simulink model "jointsControl"  (Simulink 9.1)
settings: Solver=FixedStepDiscrete  StartTime=0.0  StopTime=Config.SIMULATION_TIME  FixedStep=Config.tStep  RelTol=1e-3  EnableMultiTasking=on
PostLoadFcn:
  | %% Try to open the static GUI
  | try
  | 
  |     staticGUI = simulinkStaticGUI;
  | 
  | end
InitFcn:
  | %% initialize the simulation
  | cd(fileparts(which(bdroot)));
  | initJointsControl;
  | 
  | %% Try to edit the GUI (the user may have already closed it)
  | try
  | 
  |     %% Update Start Button
  |     set(sl_synch_handles.startButton,'Backgroundcolor',[0.0,1.0,0.0]);
  |     set(sl_synch_handles.startButton,'Enable','on');
  | 
  | end
StartFcn:
  | %% Try to edit the GUI (the user may have already closed it)
  | try
  | 
  |     %% Update Start Button
  |     set(sl_synch_handles.startButton,'Backgroundcolor',[0.8,0.8,0.8]);
  |     set(sl_synch_handles.startButton,'Enable','off');
  | 
  |     %% Update Compile Button
  |     set(sl_synch_handles.compileButton,'Backgroundcolor',[0.8,0.8,0.8]);
  |     set(sl_synch_handles.compileButton,'Enable','off');
  | 
  |     %% Update Exit Button
  |     set(sl_synch_handles.exitButton,'Backgroundcolor',[0.8,0.8,0.8]);
  |     set(sl_synch_handles.exitButton,'Enable','off');
  | 
  | end
StopFcn:
  | %% stop the simulation
  | cd(fileparts(which(bdroot)));
  | stopJointsControl;
  | 
  | %% Try to edit the GUI (the user may have already closed it)
  | try
  | 
  |     %% Update Compile Button
  |     set(sl_synch_handles.compileButton,'Backgroundcolor',[1.0,0.6,0.0]);
  |     set(sl_synch_handles.compileButton,'Enable','on');
  | 
  |     %% Update Exit Button
  |     set(sl_synch_handles.exitButton,'Backgroundcolor',[0.0,1.0,1.0]);
  |     set(sl_synch_handles.exitButton,'Enable','on');
  | 
  | end
undefined symbols (not defined in the file): Config, KD, KP, Ref, ROBOT_DOF, Sat
libraries: WBToolboxLibrary x12
CloseFcn:
  | %% Try to close the GUI (the user might have already closed it)
  | try
  | 
  |     close(simulinkStaticGUI)
  | 
  | end
settings Model: SuppressorTable=22 serialization::archive 11 0 6 0 0 0 1 0  Creator=daniele  LastModifiedBy=icub
settings DataIOCC: LimitDataPoints=on  SignalLoggingSaveFormat=ModelDataLogs
settings DebuggingCC: UnderspecifiedInitializationDetection=Simplified  MergeDetectMultiDrivingBlocksExec=error  SolverPrmCheckMsg=warning  MultiTaskDSMMsg=warning  MultiTaskCondExecSysMsg=none  AllowSymbolicDim=off  StrictBusMsg=ErrorOnBusTreatedAsVector
settings GRTTargetCC: GeneratePreprocessorConditionals=Disable all  CombineOutputUpdateFcns=on  GRTInterface=off

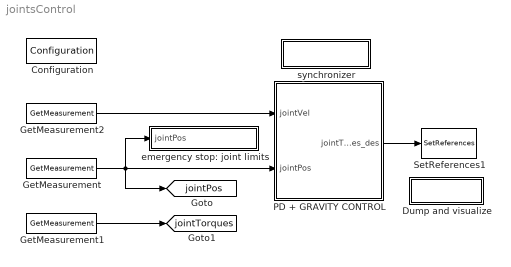
== system jointsControl ==
  Configuration : WBToolboxLibrary/Utilities/Configuration  ConfigSource=Workspace  ConfigObject='WBTConfigRobot'
      settings: SourceProductName=WholeBodyToolbox
  Dump and visualize : Subsystem
      mask Display: disp('VISUALIZER')
  GetMeasurement : WBToolboxLibrary/States/GetMeasurement  measuredType=Joints Position
      settings: SourceProductName=WholeBodyToolbox
  GetMeasurement1 : WBToolboxLibrary/States/GetMeasurement  measuredType=Joints Torque
      settings: SourceProductName=WholeBodyToolbox
  GetMeasurement2 : WBToolboxLibrary/States/GetMeasurement  measuredType=Joints Velocity
      settings: SourceProductName=WholeBodyToolbox
  PD + GRAVITY CONTROL : Subsystem
  SetReferences1 : WBToolboxLibrary/Actuators/SetReferences  controlType=Torque  refSpeed=50  refAcceleration=1000000*(pi/180)
      settings: SourceProductName=WholeBodyToolbox
  emergency stop: joint limits : Subsystem
      mask Display: disp('EMERGENCY STOP')
  synchronizer : Subsystem
      mask Display: disp('SYNCHRONIZER')
  tag scope: jointPos=global, jointTorques=global
  wires:
  GetMeasurement/1 -> [jointPos], emergency stop: joint limits/1(jointPos), PD + GRAVITY CONTROL/2(jointPos)
  PD + GRAVITY CONTROL/1(jointTorques_des) -> SetReferences1/1
  GetMeasurement2/1 -> PD + GRAVITY CONTROL/1(jointVel)
  GetMeasurement1/1 -> [jointTorques]

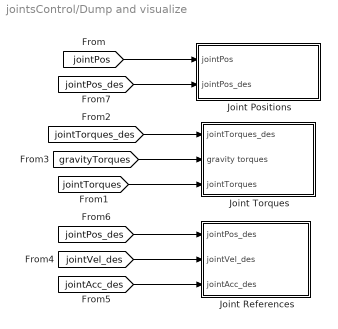
== system jointsControl/Dump and visualize ==
  Joint Positions : Subsystem
  Joint References : Subsystem
  Joint Torques : Subsystem
  wires:
  [jointTorques] -> Joint Torques/3(jointTorques)
  [gravityTorques] -> Joint Torques/2(gravity torques)
  [jointTorques_des] -> Joint Torques/1(jointTorques_des)
  [jointPos] -> Joint Positions/1(jointPos)
  [jointPos_des] -> Joint References/1(jointPos_des)
  [jointVel_des] -> Joint References/2(jointVel_des)
  [jointAcc_des] -> Joint References/3(jointAcc_des)
  [jointPos_des] -> Joint Positions/2(jointPos_des)

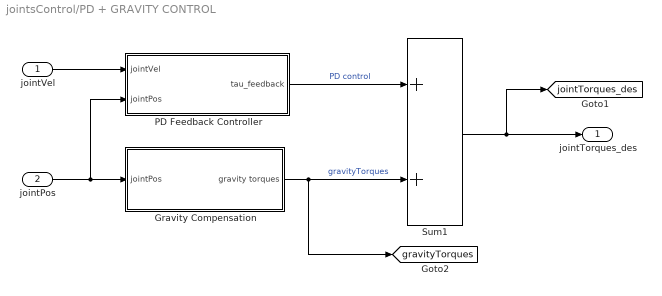
== system jointsControl/PD + GRAVITY CONTROL ==
  jointVel : Inport
  jointPos : Inport  Port=2
  Gravity Compensation : Subsystem
  PD Feedback Controller : Subsystem
  Sum1 : Sum
  jointTorques_des : Outport
  tag scope: gravityTorques=global, jointTorques_des=global
  wires:
  jointPos/1 -> PD Feedback Controller/2(jointPos), Gravity Compensation/1(jointPos)
  jointVel/1 -> PD Feedback Controller/1(jointVel)
  Sum1/1 -> [jointTorques_des], jointTorques_des/1
  Gravity Compensation/1(gravity torques) -> [gravityTorques], Sum1/2  "gravityTorques"
  PD Feedback Controller/1(tau_feedback) -> Sum1/1  "PD control"

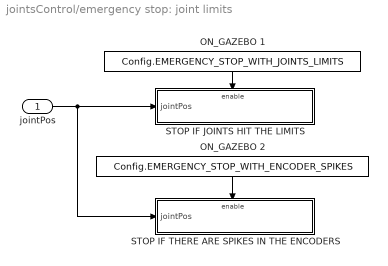
== system jointsControl/emergency stop: joint limits ==
  jointPos : Inport
  ON_GAZEBO 1 : Constant  Value=Config.EMERGENCY_STOP_WITH_JOINTS_LIMITS
  ON_GAZEBO 2 : Constant  Value=Config.EMERGENCY_STOP_WITH_ENCODER_SPIKES
  STOP IF JOINTS HIT THE LIMITS : Subsystem
  STOP IF THERE ARE SPIKES IN THE ENCODERS : Subsystem
  wires:
  ON_GAZEBO 1/1 -> STOP IF JOINTS HIT THE LIMITS/Enable
  jointPos/1 -> STOP IF THERE ARE SPIKES IN THE ENCODERS/1(jointPos), STOP IF JOINTS HIT THE LIMITS/1(jointPos)
  ON_GAZEBO 2/1 -> STOP IF THERE ARE SPIKES IN THE ENCODERS/Enable

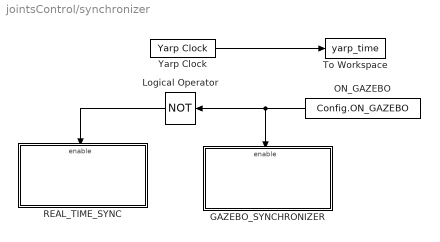
== system jointsControl/synchronizer ==
  GAZEBO_SYNCHRONIZER : Subsystem
  Logical Operator : Logic  Operator=NOT  AllPortsSameDT=off  OutDataTypeStr=boolean
  "ON_GAZEBO " : Constant  Value=Config.ON_GAZEBO
  REAL_TIME_SYNC : Subsystem
  To Workspace : ToWorkspace  VariableName=yarp_time  SaveFormat=Structure With Time  SampleTime=-1
  Yarp Clock : WBToolboxLibrary/Utilities/Yarp Clock
      settings: SourceProductName=WholeBodyToolbox
  wires:
  Logical Operator/1 -> REAL_TIME_SYNC/Enable
  "ON_GAZEBO "/1 -> GAZEBO_SYNCHRONIZER/Enable, Logical Operator/1
  Yarp Clock/1 -> To Workspace/1

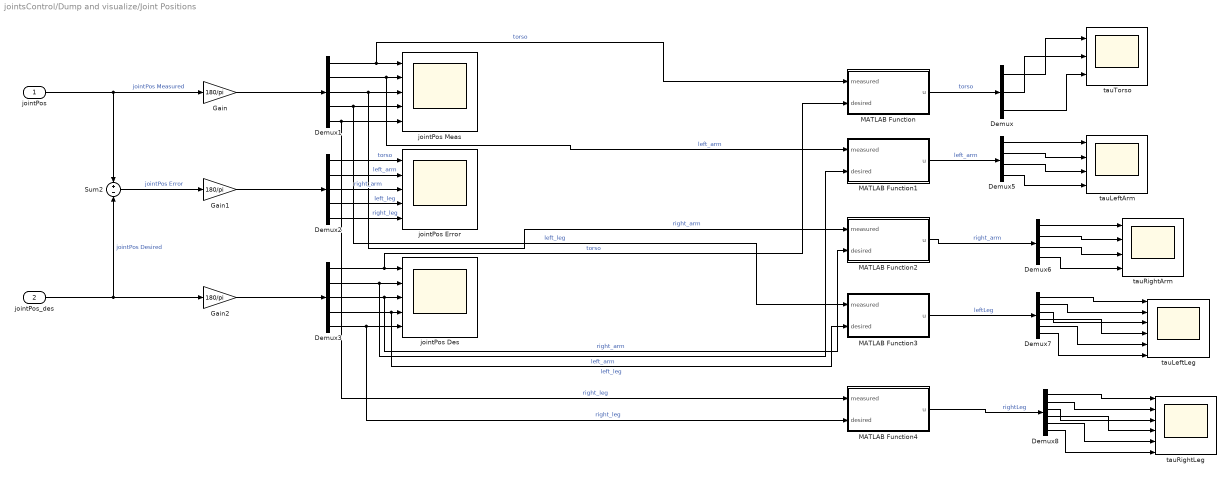
== system jointsControl/Dump and visualize/Joint Positions ==
  jointPos : Inport
  jointPos_des : Inport  Port=2
  Demux : Demux  Outputs=[2 2 2]
  Demux1 : Demux  Outputs=Config.numOfJointsForEachControlboard
  Demux2 : Demux  Outputs=Config.numOfJointsForEachControlboard
  Demux3 : Demux  Outputs=Config.numOfJointsForEachControlboard
  Demux5 : Demux  Outputs=[2 2 2 2]
  Demux6 : Demux  Outputs=[2 2 2 2]
  Demux7 : Demux  Outputs=[2 2 2 2 2 2]
  Demux8 : Demux  Outputs=[2 2 2 2 2 2]
  Gain : Gain  Gain=180/pi
  Gain1 : Gain  Gain=180/pi
  Gain2 : Gain  Gain=180/pi
  MATLAB Function : MATLAB Function  TreatAsAtomicUnit=on
  MATLAB Function1 : MATLAB Function  TreatAsAtomicUnit=on
  MATLAB Function2 : MATLAB Function  TreatAsAtomicUnit=on
  MATLAB Function3 : MATLAB Function  TreatAsAtomicUnit=on
  MATLAB Function4 : MATLAB Function  TreatAsAtomicUnit=on
  Sum2 : Sum  Inputs=+|-
  jointPos Des : Scope  NumInputPorts=5
  jointPos Error : Scope  NumInputPorts=5
  jointPos Meas : Scope  NumInputPorts=5
  tauLeftArm : Scope  NumInputPorts=4
  tauLeftLeg : Scope  NumInputPorts=6
  tauRightArm : Scope  NumInputPorts=4
  tauRightLeg : Scope  NumInputPorts=6
  tauTorso : Scope  NumInputPorts=3
  wires:
  jointPos/1 -> Sum2/1, Gain/1  "jointPos Measured"
  Demux1/2 -> MATLAB Function1/1(measured), jointPos Meas/2  "left_arm"
  Demux1/4 -> MATLAB Function3/1(measured), jointPos Meas/4  "left_leg"
  Demux1/3 -> MATLAB Function2/1(measured), jointPos Meas/3  "right_arm"
  Demux1/5 -> MATLAB Function4/1(measured), jointPos Meas/5  "right_leg"
  Demux2/1 -> jointPos Error/1  "torso"
  Demux2/2 -> jointPos Error/2  "left_arm"
  Demux2/4 -> jointPos Error/4  "left_leg"
  Demux2/3 -> jointPos Error/3  "right_arm"
  Demux2/5 -> jointPos Error/5  "right_leg"
  Sum2/1 -> Gain1/1  "jointPos Error"
  Demux3/1 -> MATLAB Function/2(desired), jointPos Des/1  "torso"
  Demux3/2 -> MATLAB Function1/2(desired), jointPos Des/2  "left_arm"
  Demux3/4 -> MATLAB Function3/2(desired), jointPos Des/4  "left_leg"
  Demux3/3 -> MATLAB Function2/2(desired), jointPos Des/3  "right_arm"
  jointPos_des/1 -> Gain2/1, Sum2/2  "jointPos Desired"
  Demux3/5 -> MATLAB Function4/2(desired), jointPos Des/5  "right_leg"
  Gain/1 -> Demux1/1
  Gain1/1 -> Demux2/1
  Gain2/1 -> Demux3/1
  MATLAB Function4/1(u) -> Demux8/1  "rightLeg"
  Demux5/1 -> tauLeftArm/1
  Demux7/3 -> tauLeftLeg/3
  Demux7/4 -> tauLeftLeg/4
  Demux7/5 -> tauLeftLeg/5
  Demux5/2 -> tauLeftArm/2
  Demux7/1 -> tauLeftLeg/1
  MATLAB Function/1(u) -> Demux/1  "torso"
  Demux6/2 -> tauRightArm/2
  Demux8/4 -> tauRightLeg/4
  Demux6/3 -> tauRightArm/3
  Demux5/4 -> tauLeftArm/4
  Demux1/1 -> MATLAB Function/1(measured), jointPos Meas/1  "torso"
  Demux6/1 -> tauRightArm/1
  MATLAB Function2/1(u) -> Demux6/1  "right_arm"
  Demux/1 -> tauTorso/1
  Demux7/6 -> tauLeftLeg/6
  Demux/2 -> tauTorso/2
  Demux8/1 -> tauRightLeg/1
  Demux6/4 -> tauRightArm/4
  Demux5/3 -> tauLeftArm/3
  Demux/3 -> tauTorso/3
  Demux8/6 -> tauRightLeg/6
  Demux8/5 -> tauRightLeg/5
  MATLAB Function3/1(u) -> Demux7/1  "leftLeg"
  Demux7/2 -> tauLeftLeg/2
  Demux8/2 -> tauRightLeg/2
  MATLAB Function1/1(u) -> Demux5/1  "left_arm"
  Demux8/3 -> tauRightLeg/3

== system jointsControl/Dump and visualize/Joint References ==
  jointPos_des : Inport
  jointVel_des : Inport  Port=2
  jointAcc_des : Inport  Port=3
  Visualize References : Scope  NumInputPorts=3
  wires:
  jointAcc_des/1 -> Visualize References/3
  jointVel_des/1 -> Visualize References/2
  jointPos_des/1 -> Visualize References/1

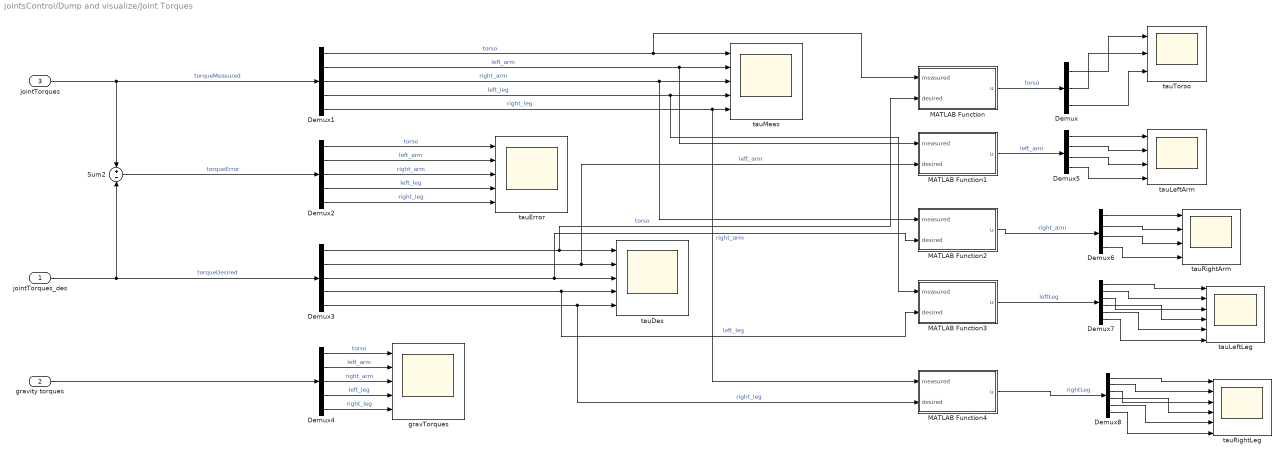
== system jointsControl/Dump and visualize/Joint Torques ==
  jointTorques_des : Inport
  gravity torques : Inport  Port=2
  jointTorques : Inport  Port=3
  Demux : Demux  Outputs=[2 2 2]
  Demux{1..4} (4 alike) : Demux  Outputs=Config.numOfJointsForEachControlboard
  Demux5 : Demux  Outputs=[2 2 2 2]
  Demux6 : Demux  Outputs=[2 2 2 2]
  Demux7 : Demux  Outputs=[2 2 2 2 2 2]
  Demux8 : Demux  Outputs=[2 2 2 2 2 2]
  MATLAB Function : MATLAB Function  TreatAsAtomicUnit=on
  MATLAB Function1 : MATLAB Function  TreatAsAtomicUnit=on
  MATLAB Function2 : MATLAB Function  TreatAsAtomicUnit=on
  MATLAB Function3 : MATLAB Function  TreatAsAtomicUnit=on
  MATLAB Function4 : MATLAB Function  TreatAsAtomicUnit=on
  Sum2 : Sum  Inputs=+|-
  gravTorques : Scope  NumInputPorts=5
  tauDes : Scope  NumInputPorts=5
  tauError : Scope  NumInputPorts=5
  tauLeftArm : Scope  NumInputPorts=4
  tauLeftLeg : Scope  NumInputPorts=6
  tauMeas : Scope  NumInputPorts=5
  tauRightArm : Scope  NumInputPorts=4
  tauRightLeg : Scope  NumInputPorts=6
  tauTorso : Scope  NumInputPorts=3
  wires:
  gravity torques/1 -> Demux4/1
  jointTorques/1 -> Demux1/1, Sum2/1  "torqueMeasured"
  Demux1/1 -> MATLAB Function/1(measured), tauMeas/1  "torso"
  Demux1/2 -> MATLAB Function1/1(measured), tauMeas/2  "left_arm"
  Demux1/4 -> MATLAB Function3/1(measured), tauMeas/4  "left_leg"
  Demux1/3 -> MATLAB Function2/1(measured), tauMeas/3  "right_arm"
  Demux1/5 -> MATLAB Function4/1(measured), tauMeas/5  "right_leg"
  Demux2/1 -> tauError/1  "torso"
  Demux2/2 -> tauError/2  "left_arm"
  Demux2/4 -> tauError/4  "left_leg"
  Demux2/3 -> tauError/3  "right_arm"
  Demux2/5 -> tauError/5  "right_leg"
  Sum2/1 -> Demux2/1  "torqueError"
  Demux3/1 -> MATLAB Function/2(desired), tauDes/1  "torso"
  Demux3/2 -> MATLAB Function1/2(desired), tauDes/2  "left_arm"
  Demux3/4 -> MATLAB Function3/2(desired), tauDes/4  "left_leg"
  Demux3/3 -> MATLAB Function2/2(desired), tauDes/3  "right_arm"
  jointTorques_des/1 -> Demux3/1, Sum2/2  "torqueDesired"
  Demux3/5 -> MATLAB Function4/2(desired), tauDes/5  "right_leg"
  Demux4/1 -> gravTorques/1  "torso"
  Demux4/2 -> gravTorques/2  "left_arm"
  Demux4/4 -> gravTorques/4  "left_leg"
  Demux4/3 -> gravTorques/3  "right_arm"
  Demux4/5 -> gravTorques/5  "right_leg"
  MATLAB Function/1(u) -> Demux/1  "torso"
  Demux/1 -> tauTorso/1
  Demux/2 -> tauTorso/2
  Demux/3 -> tauTorso/3
  MATLAB Function1/1(u) -> Demux5/1  "left_arm"
  Demux5/1 -> tauLeftArm/1
  Demux5/2 -> tauLeftArm/2
  Demux5/3 -> tauLeftArm/3
  Demux5/4 -> tauLeftArm/4
  Demux6/4 -> tauRightArm/4
  Demux6/3 -> tauRightArm/3
  Demux6/2 -> tauRightArm/2
  Demux6/1 -> tauRightArm/1
  MATLAB Function2/1(u) -> Demux6/1  "right_arm"
  MATLAB Function3/1(u) -> Demux7/1  "leftLeg"
  Demux7/1 -> tauLeftLeg/1
  Demux7/2 -> tauLeftLeg/2
  Demux7/3 -> tauLeftLeg/3
  Demux7/4 -> tauLeftLeg/4
  Demux7/5 -> tauLeftLeg/5
  Demux7/6 -> tauLeftLeg/6
  Demux8/6 -> tauRightLeg/6
  Demux8/5 -> tauRightLeg/5
  Demux8/4 -> tauRightLeg/4
  Demux8/3 -> tauRightLeg/3
  Demux8/2 -> tauRightLeg/2
  Demux8/1 -> tauRightLeg/1
  MATLAB Function4/1(u) -> Demux8/1  "rightLeg"

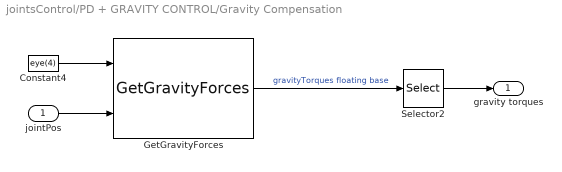
== system jointsControl/PD + GRAVITY CONTROL/Gravity Compensation ==
  jointPos : Inport
  Constant4 : Constant  Value=eye(4)
  GetGravityForces : WBToolboxLibrary/Model/Dynamics/GetGravityForces
      settings: SourceProductName=WholeBodyToolbox
  Selector2 : Selector  InputPortWidth=ROBOT_DOF+6  IndexOptions=Index vector (dialog)  Indices=[7:ROBOT_DOF+6]  OutputSizes=1
  gravity torques : Outport
  wires:
  Selector2/1 -> gravity torques/1
  Constant4/1 -> GetGravityForces/1
  jointPos/1 -> GetGravityForces/2
  GetGravityForces/1 -> Selector2/1  "gravityTorques floating base"

== system jointsControl/PD + GRAVITY CONTROL/PD Feedback Controller ==
  jointVel : Inport
  jointPos : Inport  Port=2
  PD Controller : Subsystem
  Reference Generator : Subsystem
  tau_feedback : Outport
  wires:
  jointVel/1 -> PD Controller/4(jointVel)
  jointPos/1 -> Reference Generator/1(jointPos), PD Controller/5(jointPos)
  PD Controller/1(tau_feedback) -> tau_feedback/1
  Reference Generator/1(Ms*jointAcc_des) -> PD Controller/1(Ms*jointAcc_des)
  Reference Generator/2(jointPos_des) -> PD Controller/2(jointPos_des)
  Reference Generator/3(jointVel_des) -> PD Controller/3(jointVel_des)

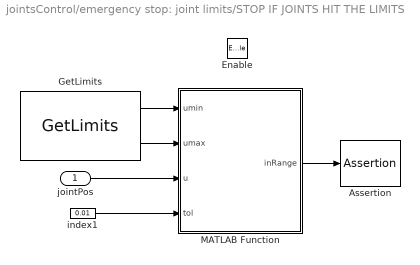
== system jointsControl/emergency stop: joint limits/STOP IF JOINTS HIT THE LIMITS ==
  jointPos : Inport
  Enable : EnablePort
  Assertion : Assertion
  GetLimits : WBToolboxLibrary/States/GetLimits  limitsSource=ControlBoard  limitsType=Position
      settings: SourceProductName=WholeBodyToolbox
  MATLAB Function : MATLAB Function  TreatAsAtomicUnit=on
  index1 : Constant  Value=0.01  VectorParams1D=off
  wires:
  jointPos/1 -> MATLAB Function/3(u)
  MATLAB Function/1(inRange) -> Assertion/1
  GetLimits/1 -> MATLAB Function/1(umin)
  GetLimits/2 -> MATLAB Function/2(umax)
  index1/1 -> MATLAB Function/4(tol)

== system jointsControl/emergency stop: joint limits/STOP IF THERE ARE SPIKES IN THE ENCODERS ==
  jointPos : Inport
  Enable : EnablePort
  Assertion : Assertion
  MATLAB Function : MATLAB Function  TreatAsAtomicUnit=on
  index1 : Constant  Value=Sat.maxJointsPositionDelta  VectorParams1D=off
  wires:
  jointPos/1 -> MATLAB Function/1(u)
  MATLAB Function/1(noSpikes) -> Assertion/1
  index1/1 -> MATLAB Function/2(delta_u_max)

== system jointsControl/synchronizer/GAZEBO_SYNCHRONIZER ==
  Enable : EnablePort
  Simulator Synchronizer : WBToolboxLibrary/Utilities/Simulator Synchronizer  period=Config.tStep  serverPortName='/clock/rpc'  clientPortName='/WBT_synchronizer/rpc:o'
      settings: SourceProductName=WholeBodyToolbox

== system jointsControl/synchronizer/REAL_TIME_SYNC ==
  Enable : EnablePort
  Real Time Synchronizer : WBToolboxLibrary/Utilities/Real Time Synchronizer  period=Config.tStep
      settings: SourceProductName=WholeBodyToolbox

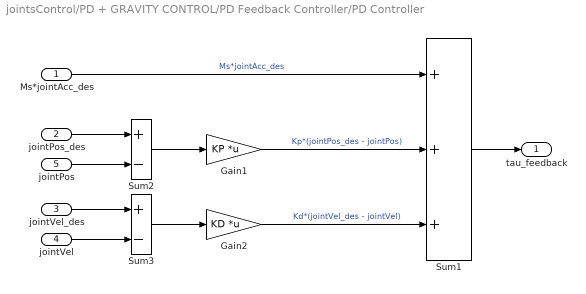
== system jointsControl/PD + GRAVITY CONTROL/PD Feedback Controller/PD Controller ==
  Ms*jointAcc_des : Inport
  jointPos_des : Inport  Port=2
  jointVel_des : Inport  Port=3
  jointVel : Inport  Port=4
  jointPos : Inport  Port=5
  Gain1 : Gain  Gain=KP  Multiplication=Matrix(K*u)
  Gain2 : Gain  Gain=KD  Multiplication=Matrix(K*u)
  Sum1 : Sum  Inputs=+++
  Sum2 : Sum  Inputs=+-
  Sum3 : Sum  Inputs=+-
  tau_feedback : Outport
  wires:
  Gain2/1 -> Sum1/3  "Kd*(jointVel_des - jointVel)"
  Sum2/1 -> Gain1/1
  jointVel/1 -> Sum3/2
  Gain1/1 -> Sum1/2  "Kp*(jointPos_des - jointPos)"
  jointPos_des/1 -> Sum2/1
  Sum3/1 -> Gain2/1
  Ms*jointAcc_des/1 -> Sum1/1  "Ms*jointAcc_des"
  Sum1/1 -> tau_feedback/1
  jointPos/1 -> Sum2/2
  jointVel_des/1 -> Sum3/1

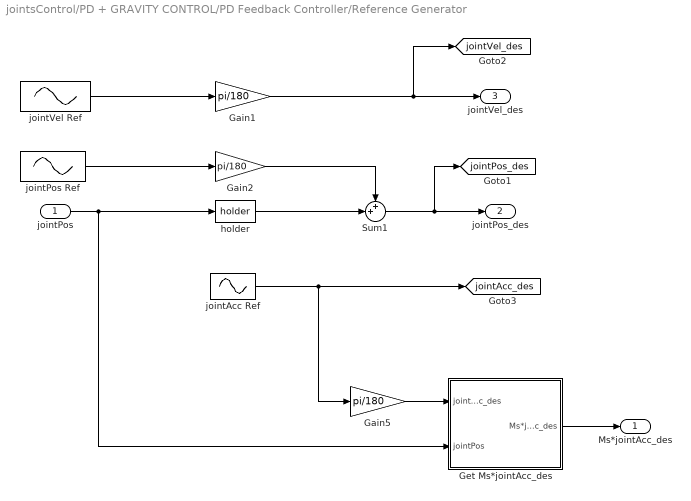
== system jointsControl/PD + GRAVITY CONTROL/PD Feedback Controller/Reference Generator ==
  jointPos : Inport
  Gain1 : Gain  Gain=pi/180
  Gain2 : Gain  Gain=pi/180
  Gain5 : Gain  Gain=pi/180
  Get Ms*jointAcc_des : Subsystem
  Sum1 : Sum  Inputs=++|
  holder : WBToolboxLibrary/Utilities/holder 
      settings: SourceProductName=WholeBodyToolbox
  jointAcc Ref : Sin  Amplitude=-Ref.Amplitude.*(Ref.Frequency.*2.*pi).^2  Frequency=Ref.Frequency.*2.*pi  SampleTime=0
  jointPos Ref : Sin  Amplitude=Ref.Amplitude  Frequency=Ref.Frequency.*2.*pi  SampleTime=0
  jointVel Ref : Sin  Amplitude=Ref.Amplitude.*Ref.Frequency.*2.*pi  Frequency=Ref.Frequency.*2.*pi  Phase=pi/2  SampleTime=0
  Ms*jointAcc_des : Outport
  jointPos_des : Outport  Port=2
  jointVel_des : Outport  Port=3
  tag scope: jointAcc_des=global, jointPos_des=global, jointVel_des=global
  wires:
  jointPos/1 -> holder/1, Get Ms*jointAcc_des/2(jointPos)
  Sum1/1 -> [jointPos_des], jointPos_des/1
  Get Ms*jointAcc_des/1(Ms*jointAcc_des) -> Ms*jointAcc_des/1
  Gain5/1 -> Get Ms*jointAcc_des/1(jointAcc_des)
  jointPos Ref/1 -> Gain2/1
  jointVel Ref/1 -> Gain1/1
  Gain1/1 -> [jointVel_des], jointVel_des/1
  jointAcc Ref/1 -> Gain5/1, [jointAcc_des]
  Gain2/1 -> Sum1/1
  holder/1 -> Sum1/2

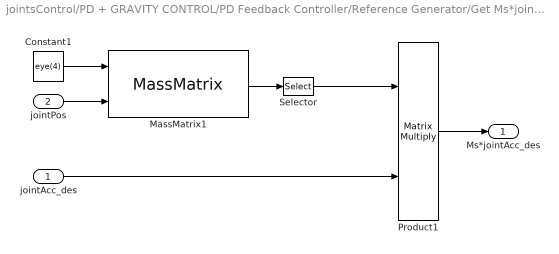
== system jointsControl/PD + GRAVITY CONTROL/PD Feedback Controller/Reference Generator/Get Ms*jointAcc_des ==
  jointAcc_des : Inport
  jointPos : Inport  Port=2
  Constant1 : Constant  Value=eye(4)
  MassMatrix1 : WBToolboxLibrary/Model/Dynamics/MassMatrix
      settings: SourceProductName=WholeBodyToolbox
  Product1 : Product  Multiplication=Matrix(*)
  Selector : Selector  NumberOfDimensions=2  InputPortWidth=3  IndexOptions=Index vector (dialog),Index vector (dialog)  Indices=[7:ROBOT_DOF+6],[7:ROBOT_DOF+6]  OutputSizes=1,1
  Ms*jointAcc_des : Outport
  wires:
  MassMatrix1/1 -> Selector/1
  Product1/1 -> Ms*jointAcc_des/1
  Selector/1 -> Product1/1
  Constant1/1 -> MassMatrix1/1
  jointPos/1 -> MassMatrix1/2
  jointAcc_des/1 -> Product1/2

== matlab function Dump and visualize/Joint Torques/MATLAB Function1 ==
  data: measured input double; u output double; desired input double
function u = fcn(measured, desired)


u = zeros(1, length(measured) + length(desired))';

j = 1;
for i =1:length(measured)
   u(j) = desired(i);
   j = j+1;
   u(j) = measured(i);
   j = j+1;
end

== matlab function Dump and visualize/Joint Torques/MATLAB Function ==
  data: measured input double; u output double; desired input double
function u = fcn(measured, desired)


u = zeros(1, length(measured) + length(desired))';

j = 1;
for i =1:length(measured)
   u(j) = desired(i);
   j = j+1;
   u(j) = measured(i);
   j = j+1;
end

== matlab function Dump and visualize/Joint Torques/MATLAB Function2 ==
  data: measured input double; u output double; desired input double
function u = fcn(measured, desired)


u = zeros(1, length(measured) + length(desired))';

j = 1;
for i =1:length(measured)
   u(j) = desired(i);
   j = j+1;
   u(j) = measured(i);
   j = j+1;
end

== matlab function Dump and visualize/Joint Torques/MATLAB Function3 ==
  data: measured input double; u output double; desired input double
function u = fcn(measured, desired)


u = zeros(1, length(measured) + length(desired))';

j = 1;
for i =1:length(measured)
   u(j) = desired(i);
   j = j+1;
   u(j) = measured(i);
   j = j+1;
end

== matlab function Dump and visualize/Joint Torques/MATLAB Function4 ==
  data: measured input double; u output double; desired input double
function u = fcn(measured, desired)


u = zeros(1, length(measured) + length(desired))';

j = 1;
for i =1:length(measured)
   u(j) = desired(i);
   j = j+1;
   u(j) = measured(i);
   j = j+1;
end

== matlab function Dump and visualize/Joint Positions/MATLAB Function ==
  data: measured input double; u output double; desired input double
function u = fcn(measured, desired)


u = zeros(1, length(measured) + length(desired))';

j = 1;
for i =1:length(measured)
   u(j) = desired(i);
   j = j+1;
   u(j) = measured(i);
   j = j+1;
end

== matlab function Dump and visualize/Joint Positions/MATLAB Function1 ==
  data: measured input double; u output double; desired input double
function u = fcn(measured, desired)


u = zeros(1, length(measured) + length(desired))';

j = 1;
for i =1:length(measured)
   u(j) = desired(i);
   j = j+1;
   u(j) = measured(i);
   j = j+1;
end

== matlab function Dump and visualize/Joint Positions/MATLAB Function2 ==
  data: measured input double; u output double; desired input double
function u = fcn(measured, desired)


u = zeros(1, length(measured) + length(desired))';

j = 1;
for i =1:length(measured)
   u(j) = desired(i);
   j = j+1;
   u(j) = measured(i);
   j = j+1;
end

== matlab function Dump and visualize/Joint Positions/MATLAB Function3 ==
  data: measured input double; u output double; desired input double
function u = fcn(measured, desired)


u = zeros(1, length(measured) + length(desired))';

j = 1;
for i =1:length(measured)
   u(j) = desired(i);
   j = j+1;
   u(j) = measured(i);
   j = j+1;
end

== matlab function Dump and visualize/Joint Positions/MATLAB Function4 ==
  data: measured input double; u output double; desired input double
function u = fcn(measured, desired)


u = zeros(1, length(measured) + length(desired))';

j = 1;
for i =1:length(measured)
   u(j) = desired(i);
   j = j+1;
   u(j) = measured(i);
   j = j+1;
end

== matlab function emergency stop: joint limits/STOP IF THERE ARE SPIKES IN THE ENCODERS/MATLAB Function ==
  data: u input double; delta_u_max input double; noSpikes output double
function noSpikes = checkSpikes(u, delta_u_max)

     noSpikes = wbc.checkSpikes(u, delta_u_max);
end

== matlab function emergency stop: joint limits/STOP IF JOINTS HIT THE LIMITS/MATLAB Function ==
  data: umin input double; umax input double; u input double; inRange output double; tol input double
function inRange = checkRangeFCN(umin, umax, u, tol)

     inRange = wbc.checkRange(umin, umax, u, tol);
end
